simulink model "SimplificationDemo_After"  (Simulink 7.8)
settings: Solver=ode45  StartTime=0.0  StopTime=10.0  RelTol=1e-3
settings Model: Creator=760162  LastModifiedBy=monika

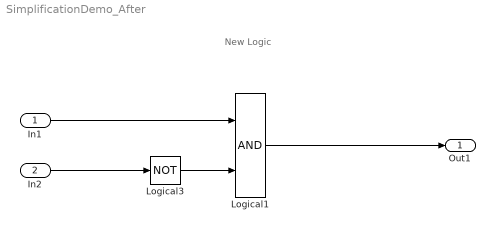
== system SimplificationDemo_After ==
  note: New Logic
  In1 : Inport
  In2 : Inport  Port=2
  Logical1 : Logic  OutDataTypeStr=boolean
  Logical3 : Logic  Operator=NOT  OutDataTypeStr=boolean
  Out1 : Outport
  wires:
  Logical3/1 -> Logical1/2
  In2/1 -> Logical3/1
  In1/1 -> Logical1/1
  Logical1/1 -> Out1/1
